simulink subsystem "Subsystem_BA_Controller"  (R2023b)
settings: Solver=VariableStepAuto  StartTime=0.0  StopTime=10.0  RelTol=1e-3
settings Model: Creator=Alberto  LastModifiedBy=Alberto

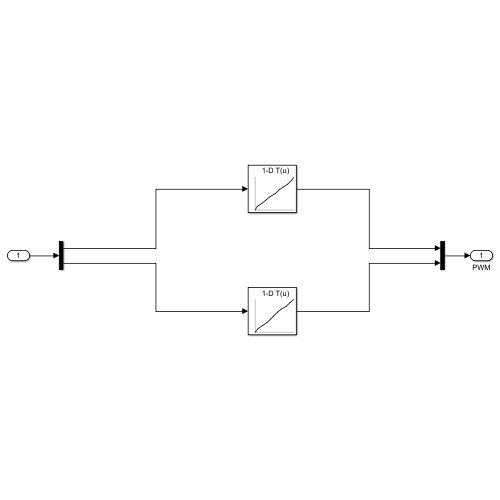
[thumbnail: Simulink's stored preview of the top-level diagram]
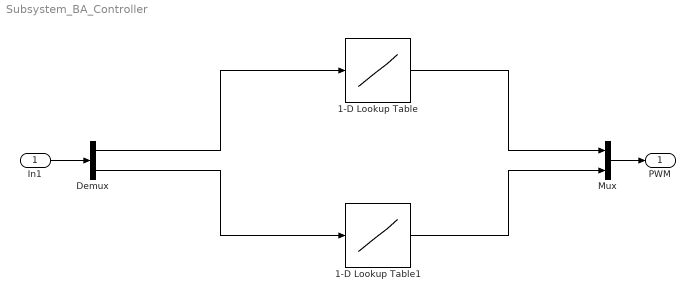
== system Subsystem_BA_Controller ==
  In1 : Inport
  1-D Lookup Table : Lookup_n-D  NumberOfTableDimensions=1  BreakpointsForDimension1=[-0.504093170166016 -0.435977935791016 -0.326982498168945 -0.231611728668213 -0.122618317604065 0 0.108993530273438 0.217994689941406 0.326980590820313 0.422355651855469 0.476848602294922]  Table=[-254 -200.660049438477 -151.130004882812 -100.32999420166 -50.8000717163086 0 51.0000114440918 100.724998474121 150.450012207031 200.175018310547 255]  InternalRulePriority=Speed  RndMeth=Simplest
  1-D Lookup Table1 : Lookup_n-D  NumberOfTableDimensions=1  BreakpointsForDimension1=[-0.461620330810547 -0.384681701660156 -0.2821044921875 -0.179512023925781 -0.076934814453125 0 0.076936960220337 0.179519176483154 0.294923782348633 0.384683609008789 0.474445343017578]  Table=[-254 -200.65998840332 -151.130004882812 -100.32999420166 -50.8000106811523 0 50.9999961853027 100.724998474121 150.450012207031 200.174987792969 255]  InternalRulePriority=Speed  RndMeth=Simplest
  Demux : Demux  Outputs=2
  Mux : Mux  Inputs=2
  PWM : Outport
  wires:
  Demux/2 -> 1-D Lookup Table1/1
  1-D Lookup Table1/1 -> Mux/2
  Mux/1 -> PWM/1
  Demux/1 -> 1-D Lookup Table/1
  In1/1 -> Demux/1
  1-D Lookup Table/1 -> Mux/1
